simulink model "ME598_R3_FinalProject_FunctionBlockAlgosFinal"  (R2021b)
settings: Solver=ode23t  StartTime=0.0  StopTime=inf  RelTol=1e-3
InitFcn:
  | RPInit
model workspace (MAT data in the model file):
  mapForSim : object (value not decoded)
  occGrid : robotics.BinaryOccupancyGrid (value not decoded)
undefined symbols (not defined in the file): X, Y, Z
libraries: sm_lib x25, nesl_utility x11, RP_Simulator_Components x7, ME598_ProjectLibrary x3, RoboticsPlayground x2, Contact_Forces_Lib x2
(part 2 of 2)

== matlab function ME598_R3_FinalProject_FunctionBlockAlgosFinal/MATLAB Function ==
  data: rDist input; gDist input; bDist input; xPose input; leftMotor output; yPose input; tPose input; left input; front input; right input; rightMotor output; inState input; tState output
function [leftMotor, rightMotor, tState] = sortDiscs(rDist, gDist, bDist, xPose, yPose, tPose, left, front, right, inState)

tState = inState;
% leftMotor = 120;
% rightMotor = 120;

    % Calculate the required angle to turn the robot to.
    function desiredAngle = calculateSlope(x1, y1, x2, y2)
        desiredAngle = atan2d(y2-y1, x2-x1);
    end

    % Motor Speeds to Turn the robot to the Right
    function [leftMotor, rightMotor] = turnRight()
        leftMotor = 60;
        rightMotor = -60;
    end
    
    % Motor Speeds to Turn the robot to the Left
    function [leftMotor, rightMotor] = turnLeft()
        leftMotor = -60;
        rightMotor = 60;
    end

    % Detect Color of the disc ahead. Only called when the disc positions
    % are reached
    function color = detectColor()
        if isnan(rDist) && isnan(gDist) && ~isnan(bDist)
            color = 'blue';
        elseif isnan(rDist) && ~isnan(gDist) && isnan(bDist)
            color = 'green';
        elseif ~isnan(rDist) && isnan(gDist) && isnan(bDist)
            color = 'red';
        else
            color = 'none';
        end
    end

    % Move the Disc to respective zone identified by 'color' variable.
    % Assuming the robot has captured the disc.
    function [leftMotor, rightMotor] = moveDiscToZone(color, nextState)
        switch color
            case 'red'
                if xPose > 1.7 && yPose > 1.7
                    leftMotor = 0;
                    rightMotor = 0;
                    tState = nextState;
                    return;
                end            
                desiredAngle = calculateSlope(xPose, yPose, 2, 2);
                [leftMotor, rightMotor] = moveRobot(desiredAngle);
            case 'blue'
                if xPose < -1.7 && yPose > -0.3 && yPose < 0.3
                    leftMotor = 0;
                    rightMotor = 0;
                    tState = nextState;
                    return;
                end            
                desiredAngle = calculateSlope(xPose, yPose, -2, 0);
                [leftMotor, rightMotor] = moveRobot(desiredAngle);
            case 'green'
                if xPose > 1.7 && yPose < -1.6
                    leftMotor = 0;
                    rightMotor = 0;
                    tState = nextState;
                    return;
                end            
                desiredAngle = calculateSlope(xPose, yPose, 2, -2);
                [leftMotor, rightMotor] = moveRobot(desiredAngle);
            otherwise 
                leftMotor = 120;
                rightMotor = 120;
        end

    end

    % Determine the robot motion. Turn or move forward.
    function [leftMotor, rightMotor] = moveRobot(desiredAngle)
        diff = tPose - desiredAngle;
        if diff > 180
            diff = diff - 360;
        elseif diff < -180
            diff = diff + 360;
        end
        if diff < -10
            [leftMotor, rightMotor] = turnLeft();
        elseif diff > 10
            [leftMotor, rightMotor] = turnRight();
        else
            leftMotor = 120;
            rightMotor = 120;
        end
    end

    % Move robot to a position. 
    function [leftMotor, rightMotor] = moveRobotToPosition(x, y, nextState)
        if xPose < x + 0.1 && xPose > x - 0.1 && yPose > y - 0.1 && yPose < y + 0.1
            leftMotor = 0;
            rightMotor = 0;
            tState = nextState;
            return;
        end
        desiredAngle = calculateSlope(xPose, yPose, x, y);
        [leftMotor, rightMotor] = moveRobot(desiredAngle);
    end

    % Get the distance of the puck.
    function dist = getPuckDistance()
        if ~isnan(rDist) && isnan(gDist) && isnan(bDist)
            dist = rDist;
        elseif isnan(rDist) && ~isnan(gDist) && isnan(bDist)
            dist = gDist;
        elseif isnan(rDist) && isnan(gDist) && ~isnan(bDist)
            dist = bDist;
        else
            dist = 10;
        end
    end

    % Move robot a bit back to free the disc/puck.
    function [leftMotor, rightMotor] = moveRobotBack(dist, nextState)
        if dist < 0.5
            leftMotor = -120;
            rightMotor = -120;
        else
            leftMotor = 0;
            rightMotor = 0;
            tState = nextState;
            return;
        end
    end

% Based on tState, determine robot actions.
switch tState
    case 0
        % Proceed to First Disc position
        [leftMotor, rightMotor] = moveRobotToPosition(0, 1.5, 1);
    
    case 1
        % Take first disc to it's home position
        color = detectColor();
        [leftMotor, rightMotor] = moveDiscToZone(color, 2);
    
    case 2
        % Move a bit back to position disc in its target zone
        dist = getPuckDistance();
        [leftMotor, rightMotor] = moveRobotBack(dist, 3);
    
    case 3
        % Proceed to second disc position
        [leftMotor, rightMotor] = moveRobotToPosition(0, -1.5, 4);

    case 4
       % Take second disc to it's home position
        color = detectColor();
        [leftMotor, rightMotor] = moveDiscToZone(color, 5);

    case 5
        % Move a bit back to position disc in its target zone
        dist = getPuckDistance();
        [leftMotor, rightMotor] = moveRobotBack(dist, 6);

    case 6
        % Move the robot back to the origin
        [leftMotor, rightMotor] = moveRobotToPosition(0, 0, 10);

    otherwise
        leftMotor = 0;
        rightMotor = 0;
end

% Wall avoidance algorithm. No matter where, if the wall is detected to be
% near, the specific robot action is triggered.
if front < 0.3
    if isnan(left) && isnan(right)
        leftMotor = -120;
        rightMotor = -120;
    elseif isnan(left) && ~isnan(right)
        [leftMotor, rightMotor] = turnLeft();
    elseif ~isnan(left) && isnan(right)
        [leftMotor, rightMotor] = turnRight();
    end
elseif right < 0.3 && isnan(left)
    [leftMotor, rightMotor] = turnLeft();
elseif left < 0.3 && isnan(right)
    [leftMotor, rightMotor] = turnRight();

end


end

== matlab function ME598_R3_FinalProject_FunctionBlockAlgosFinal/-180* : 180* ==
  data: deg input; deg output
function deg = degWrap(deg)

% % Convert radians to degrees
% deg = 180/pi * rad;


% Wrap degree value to the range -180* : +180*
for idx = 1:length(deg)
    while deg(idx) < -180
        deg(idx) = deg(idx)+360;
    end
    
    while deg(idx) > 180
        deg(idx) = deg(idx)-360;
    end
end

return
